simulink model "EJEMPLO"  (R2015a)
settings: Solver=ode45  StartTime=0.0  StopTime=0.16  RelTol=1e-3
libraries: powerlib x26
settings Model: CovSFcnEnable=off  Creator=alcaucil  LastModifiedBy=NECSOFT
settings DebuggingCC: SolverPrmCheckMsg=warning

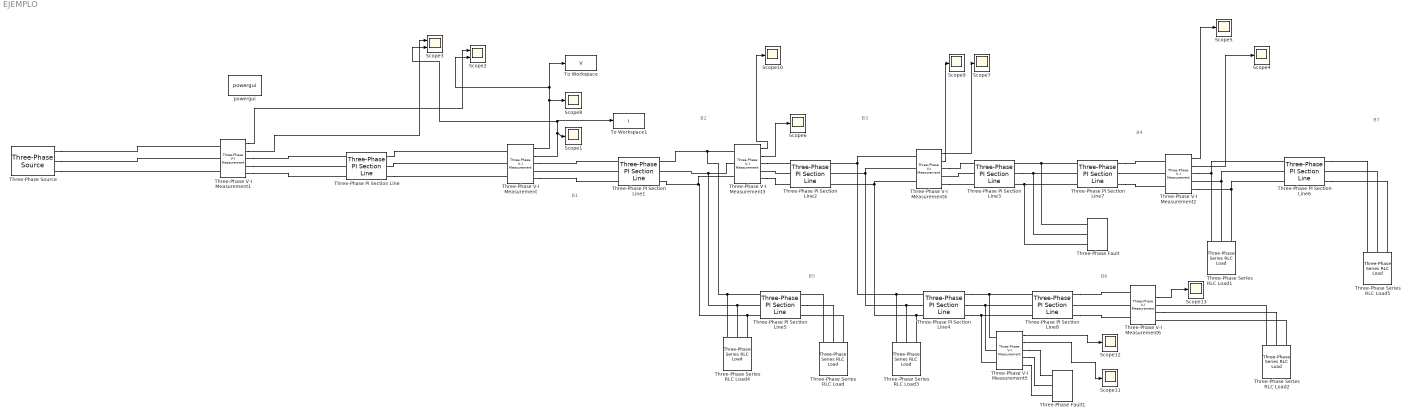
== system EJEMPLO ==
  note: B1
  note: B2
  note: B3
  note: B4
  note: B5
  note: B6
  note: B7
  Scope{1,4..13} (11 alike) : Scope
      Scope1 settings: TimeRange=0.16  YMin=-20000  YMax=20000
      Scope10 settings: YMin=-20000  YMax=20000  SaveName=ScopeData9
      Scope11 settings: YMin=-20000  YMax=20000  SaveName=ScopeData10
      Scope12 settings: YMin=-20000  YMax=20000  SaveName=ScopeData11
      Scope13 settings: YMin=-20000  YMax=20000  SaveName=ScopeData12
      Scope4 settings: YMin=-20000  YMax=20000  SaveName=ScopeData3
      Scope5 settings: YMin=-20000  YMax=20000  SaveName=ScopeData4
      Scope6 settings: YMin=-20000  YMax=20000  SaveName=ScopeData5
      Scope7 settings: YMin=-20000  YMax=20000  SaveName=ScopeData6
      Scope8 settings: YMin=-20000  YMax=20000  SaveName=ScopeData8
      Scope9 settings: YMin=-20000  YMax=20000  SaveName=ScopeData7
  Scope2 : Scope  NumInputPorts=2
      settings: YMin=-20000~-5  YMax=20000~5
  Scope3 : Scope  NumInputPorts=2
      settings: YMin=-20000~-5  YMax=20000~5  SaveName=ScopeData2
  Three-Phase PI Section Line : powerlib/Elements/Three-Phase PI Section Line  LConnTagsString=a|b|c  RConnTagsString=A|B|C  Frequency=60  Resistances=[ 0.01273 0.3864]  Inductances="[ 0.9337e-3  4.1264e-3]"  Capacitances=[7.4e-19 3.8e-19]  Length=1
  Three-Phase PI Section Line1 : powerlib/Elements/Three-Phase PI Section Line  LConnTagsString=a|b|c  RConnTagsString=A|B|C  Frequency=60  Resistances=[ 0.01273 0.3864]  Inductances="[ 0.9337e-3  4.1264e-3]"  Capacitances=[12.74e-19 7.751e-19]  Length=30
  Three-Phase PI Section Line2 : powerlib/Elements/Three-Phase PI Section Line  LConnTagsString=a|b|c  RConnTagsString=A|B|C  Frequency=60  Resistances=[ 0.01273 0.3864]  Inductances="[ 0.9337e-3  4.1264e-3]"  Capacitances=[12.74e-19 7.751e-19]  Length=15
  Three-Phase PI Section Line3 : powerlib/Elements/Three-Phase PI Section Line  LConnTagsString=a|b|c  RConnTagsString=A|B|C  Frequency=60  Resistances=[ 0.01273 0.3864]  Inductances="[ 0.9337e-3  4.1264e-3]"  Capacitances=[12.74e-19 7.751e-19]  Length=5
  Three-Phase PI Section Line4 : powerlib/Elements/Three-Phase PI Section Line  LConnTagsString=a|b|c  RConnTagsString=A|B|C  Frequency=60  Resistances=[ 0.01273 0.3864]  Inductances="[ 0.9337e-3  4.1264e-3]"  Capacitances=[12.74e-19 7.751e-19]  Length=15
  Three-Phase PI Section Line5 : powerlib/Elements/Three-Phase PI Section Line  LConnTagsString=a|b|c  RConnTagsString=A|B|C  Frequency=60  Resistances=[ 0.01273 0.3864]  Inductances="[ 0.9337e-3  4.1264e-3]"  Capacitances=[12.74e-19 7.751e-19]  Length=8
  Three-Phase PI Section Line6 : powerlib/Elements/Three-Phase PI Section Line  LConnTagsString=a|b|c  RConnTagsString=A|B|C  Frequency=60  Resistances=[ 0.01273 0.3864]  Inductances="[ 0.9337e-3  4.1264e-3]"  Capacitances=[12.74e-19 7.751e-19]  Length=19
  Three-Phase PI Section Line7 : powerlib/Elements/Three-Phase PI Section Line  LConnTagsString=a|b|c  RConnTagsString=A|B|C  Frequency=60  Resistances=[ 0.01273 0.3864]  Inductances="[ 0.9337e-3  4.1264e-3]"  Capacitances=[12.74e-19 7.751e-19]  Length=5
  Three-Phase PI Section Line8 : powerlib/Elements/Three-Phase PI Section Line  LConnTagsString=a|b|c  RConnTagsString=A|B|C  Frequency=60  Resistances=[ 0.01273 0.3864]  Inductances="[ 0.9337e-3  4.1264e-3]"  Capacitances=[12.74e-19 7.751e-19]  Length=5
  Three-Phase Series RLC Load{,1..5} (6 alike) : powerlib/Elements/Three-Phase Series RLC Load  LConnTagsString=A|B|C  Configuration=Y (grounded)  NominalVoltage=14300  NominalFrequency=60  ActivePower=8e3  InductivePower=100  CapacitivePower=0  Measurements=None  LoadType=constant Z
  Three-Phase V-I Measurement{,1..4} (5 alike) : powerlib/Measurements/Three-Phase V-I Measurement  VoltageMeasurement=phase-to-ground  SetLabelV=off  LabelV=Vabc  Vpu=off  VpuLL=off  CurrentMeasurement=yes  SetLabelI=off  LabelI=Iabc  Ipu=off  Pbase=100e6  Vbase=500e3  OutputType=Complex  PhasorSimulation=off  PSBequivalent=0
  Three-Phase V-I Measurement5 : powerlib/Measurements/Three-Phase V-I Measurement  VoltageMeasurement=phase-to-phase  SetLabelV=off  LabelV=Vabc  Vpu=off  VpuLL=off  CurrentMeasurement=yes  SetLabelI=off  LabelI=Iabc  Ipu=off  Pbase=100e6  Vbase=500e3  OutputType=Complex  PhasorSimulation=off  PSBequivalent=0
  Three-Phase V-I Measurement6 : powerlib/Measurements/Three-Phase V-I Measurement  VoltageMeasurement=phase-to-phase  SetLabelV=off  LabelV=Vabc  Vpu=off  VpuLL=off  CurrentMeasurement=yes  SetLabelI=off  LabelI=Iabc  Ipu=off  Pbase=100e6  Vbase=500e3  OutputType=Complex  PhasorSimulation=off  PSBequivalent=0
  Three-Phase Fault : powerlib/Elements/Three-Phase Fault  InitialStates=0  FaultA=off  FaultB=off  FaultC=off  GroundFault=off  SwitchTimes="[5/60  9/60]"  External=off  SwitchStatus=NaN  FaultResistance=3  GroundResistance=0.01  SnubberResistance=1e6  SnubberCapacitance=inf  Measurements=None
  Three-Phase Fault1 : powerlib/Elements/Three-Phase Fault  InitialStates=0  FaultA=on  FaultB=off  FaultC=off  GroundFault=on  SwitchTimes="[5/60  9/60]"  External=off  SwitchStatus=NaN  FaultResistance=500  GroundResistance=0.01  SnubberResistance=1e6  SnubberCapacitance=inf  Measurements=None
  Three-Phase Source : powerlib/Electrical Sources/Three-Phase Source  Voltage=14300  PhaseAngle=0  Frequency=60  InternalConnection=Yg  SpecifyImpedance=on  Resistance=0.8929  Inductance=16.58e-3  ShortCircuitLevel=100e6  BaseVoltage=115000  XRratio=7  BusType=swing  Pref=0  Qref=0  Qmin=-inf  Qmax=inf
  To Workspace : ToWorkspace  VariableName=V  SampleTime=-1
  To Workspace1 : ToWorkspace  VariableName=I  SampleTime=-1
  powergui : powerlib/powergui  Priority=1  SimulationMode=Discrete  SolverType=Tustin  SampleTime=1/(60*32)  frequency=60  SPID=off  DisableSnubberDevices=off  DisableRonSwitches=off  DisableVfSwitches=off  SwTol=0  DisplayEquations=off  Interpol=off  methode=off  Ts=0  FunctionMessages=off  echomessages=off  HookPort=off  EnableUseOfTLC=off  x0status=blocks  frequencyindice=60  Pbase=100e6  ErrMax=1e-4  Iterations=50  UnitsV=kV  UnitsW=MW  buscounter=0  RestoreLinks=warning  ResistiveCurrentMeasurement=off  Frange=[0:2:500]  Ylog=off  Xlog=on  ShowGrid=off  save=off  variable=ZData  structure=0  ZoomFFT=off  StartTime=0.0  cycles=1  DisplayStyle=1  fundamental=60  FreqAxis=off  MaxFrequency=1000  frequencyindicesteady=1  RmsSteady=1  display=off
  wires:
  Three-Phase V-I Measurement/1 -> Scope2/2, To Workspace/1, Scope8/1
  Three-Phase V-I Measurement/2 -> Scope3/2, To Workspace1/1, Scope1/1
  Three-Phase V-I Measurement1/1 -> Scope2/1
  Three-Phase V-I Measurement1/2 -> Scope3/1
  Three-Phase V-I Measurement2/2 -> Scope4/1
  Three-Phase V-I Measurement2/1 -> Scope5/1
  Three-Phase V-I Measurement3/2 -> Scope6/1
  Three-Phase V-I Measurement4/1 -> Scope7/1
  Three-Phase V-I Measurement4/2 -> Scope9/1
  Three-Phase V-I Measurement3/1 -> Scope10/1
  Three-Phase V-I Measurement5/2 -> Scope11/1
  Three-Phase V-I Measurement5/1 -> Scope12/1
  Three-Phase V-I Measurement6/2 -> Scope13/1
  connections:
  Three-Phase Series RLC Load4/LConn1 -- Three-Phase PI Section Line5/LConn1 -- Three-Phase V-I Measurement3/LConn1 -- Three-Phase PI Section Line1/RConn1
  Three-Phase PI Section Line5/LConn2 -- Three-Phase Series RLC Load4/LConn2 -- Three-Phase V-I Measurement3/LConn2 -- Three-Phase PI Section Line1/RConn2
  Three-Phase PI Section Line4/LConn1 -- Three-Phase Series RLC Load3/LConn1 -- Three-Phase V-I Measurement4/LConn1 -- Three-Phase PI Section Line2/RConn1
  Three-Phase PI Section Line4/LConn2 -- Three-Phase Series RLC Load3/LConn2 -- Three-Phase V-I Measurement4/LConn2 -- Three-Phase PI Section Line2/RConn2
  Three-Phase PI Section Line4/LConn3 -- Three-Phase Series RLC Load3/LConn3 -- Three-Phase V-I Measurement4/LConn3 -- Three-Phase PI Section Line2/RConn3
  Three-Phase Series RLC Load/LConn1 -- Three-Phase PI Section Line5/RConn1
  Three-Phase PI Section Line5/RConn2 -- Three-Phase Series RLC Load/LConn2
  Three-Phase Series RLC Load/LConn3 -- Three-Phase PI Section Line5/RConn3
  Three-Phase PI Section Line/RConn1 -- Three-Phase V-I Measurement/LConn1
  Three-Phase V-I Measurement/LConn2 -- Three-Phase PI Section Line/RConn2
  Three-Phase PI Section Line/RConn3 -- Three-Phase V-I Measurement/LConn3
  Three-Phase V-I Measurement/RConn1 -- Three-Phase PI Section Line1/LConn1
  Three-Phase PI Section Line1/LConn2 -- Three-Phase V-I Measurement/RConn2
  Three-Phase V-I Measurement/RConn3 -- Three-Phase PI Section Line1/LConn3
  Three-Phase V-I Measurement1/RConn1 -- Three-Phase PI Section Line/LConn1
  Three-Phase V-I Measurement1/RConn2 -- Three-Phase PI Section Line/LConn2
  Three-Phase V-I Measurement1/RConn3 -- Three-Phase PI Section Line/LConn3
  Three-Phase PI Section Line1/RConn3 -- Three-Phase V-I Measurement3/LConn3 -- Three-Phase PI Section Line5/LConn3 -- Three-Phase Series RLC Load4/LConn3
  Three-Phase Source/RConn3 -- Three-Phase V-I Measurement1/LConn3
  Three-Phase Source/RConn2 -- Three-Phase V-I Measurement1/LConn2
  Three-Phase Source/RConn1 -- Three-Phase V-I Measurement1/LConn1
  Three-Phase V-I Measurement2/RConn1 -- Three-Phase Series RLC Load1/LConn1 -- Three-Phase PI Section Line6/LConn1
  Three-Phase Series RLC Load1/LConn2 -- Three-Phase PI Section Line6/LConn2 -- Three-Phase V-I Measurement2/RConn2
  Three-Phase V-I Measurement2/RConn3 -- Three-Phase PI Section Line6/LConn3 -- Three-Phase Series RLC Load1/LConn3
  Three-Phase V-I Measurement3/RConn1 -- Three-Phase PI Section Line2/LConn1
  Three-Phase PI Section Line2/LConn2 -- Three-Phase V-I Measurement3/RConn2
  Three-Phase V-I Measurement3/RConn3 -- Three-Phase PI Section Line2/LConn3
  Three-Phase PI Section Line6/RConn1 -- Three-Phase Series RLC Load5/LConn1
  Three-Phase Series RLC Load5/LConn2 -- Three-Phase PI Section Line6/RConn2
  Three-Phase PI Section Line6/RConn3 -- Three-Phase Series RLC Load5/LConn3
  Three-Phase PI Section Line7/LConn1 -- Three-Phase Fault/LConn1 -- Three-Phase PI Section Line3/RConn1
  Three-Phase PI Section Line3/RConn2 -- Three-Phase Fault/LConn2 -- Three-Phase PI Section Line7/LConn2
  Three-Phase PI Section Line7/LConn3 -- Three-Phase Fault/LConn3 -- Three-Phase PI Section Line3/RConn3
  Three-Phase PI Section Line7/RConn1 -- Three-Phase V-I Measurement2/LConn1
  Three-Phase V-I Measurement2/LConn2 -- Three-Phase PI Section Line7/RConn2
  Three-Phase PI Section Line7/RConn3 -- Three-Phase V-I Measurement2/LConn3
  Three-Phase V-I Measurement4/RConn1 -- Three-Phase PI Section Line3/LConn1
  Three-Phase PI Section Line3/LConn2 -- Three-Phase V-I Measurement4/RConn2
  Three-Phase V-I Measurement4/RConn3 -- Three-Phase PI Section Line3/LConn3
  Three-Phase PI Section Line4/RConn1 -- Three-Phase V-I Measurement5/LConn1 -- Three-Phase PI Section Line8/LConn1
  Three-Phase PI Section Line8/LConn2 -- Three-Phase V-I Measurement5/LConn2 -- Three-Phase PI Section Line4/RConn2
  Three-Phase PI Section Line4/RConn3 -- Three-Phase V-I Measurement5/LConn3 -- Three-Phase PI Section Line8/LConn3
  Three-Phase V-I Measurement5/RConn1 -- Three-Phase Fault1/LConn1
  Three-Phase V-I Measurement5/RConn2 -- Three-Phase Fault1/LConn2
  Three-Phase V-I Measurement5/RConn3 -- Three-Phase Fault1/LConn3
  Three-Phase PI Section Line8/RConn1 -- Three-Phase V-I Measurement6/LConn1
  Three-Phase V-I Measurement6/LConn2 -- Three-Phase PI Section Line8/RConn2
  Three-Phase PI Section Line8/RConn3 -- Three-Phase V-I Measurement6/LConn3
  Three-Phase Series RLC Load2/LConn1 -- Three-Phase V-I Measurement6/RConn1
  Three-Phase V-I Measurement6/RConn2 -- Three-Phase Series RLC Load2/LConn2
  Three-Phase Series RLC Load2/LConn3 -- Three-Phase V-I Measurement6/RConn3
